simulink model "simple_model2"  (R2024a)
settings: Solver=VariableStepAuto  StartTime=0.0  StopTime=10.0  RelTol=1e-3
libraries: simulink x1
settings Model: Creator=tyang  LastModifiedBy=tyang

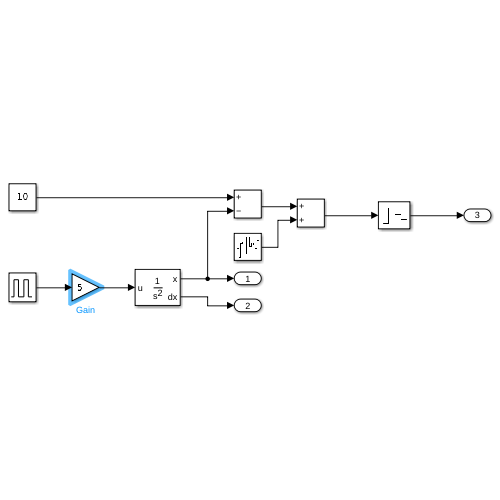
[thumbnail: Simulink's stored preview of the top-level diagram]
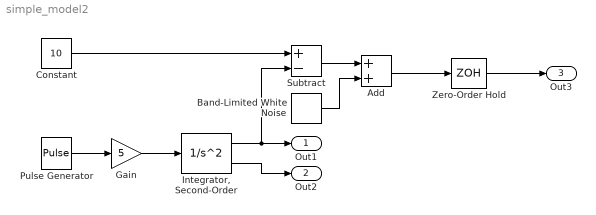
== system simple_model2 ==
  Add : Sum
  Band-Limited White Noise : simulink/Sources/Band-Limited White Noise  Cov=0.001  Ts=0.1  seed=[23341]
  Constant : Constant  Value=10
  Gain : Gain  Gain=5
  "Integrator, Second-Order" : SecondOrderIntegrator  LimitX=on  UpperLimitX=10
  Pulse Generator : DiscretePulseGenerator  PulseType=Time based  Period=10  PulseWidth=5
  Subtract : Sum  Inputs=+-
  Zero-Order Hold : ZeroOrderHold  SampleTime=0.1
  Out1 : Outport
  Out2 : Outport  Port=2
  Out3 : Outport  Port=3
  wires:
  Band-Limited White Noise/1 -> Add/2
  Subtract/1 -> Add/1
  "Integrator, Second-Order"/2 -> Out2/1
  "Integrator, Second-Order"/1 -> Subtract/2, Out1/1
  Constant/1 -> Subtract/1
  Gain/1 -> "Integrator, Second-Order"/1
  Pulse Generator/1 -> Gain/1
  Add/1 -> Zero-Order Hold/1
  Zero-Order Hold/1 -> Out3/1
